simulink model "PMSM_Drive_FastSimulation"  (R2024a)
settings: Solver=ode23t  StartTime=0.0  StopTime=0.2  FixedStep=Ts  RelTol=1e-3  AbsTol=1e-3
PreLoadFcn:
  | % Control parameters
  | Ts = 2e-6;   % Fundamental sample time
  | fsw = 2e3;   % Switching frequency (Hz)
  | fc = fsw*10; % Control loop frequency (Hz)
  | Tsc = 1/fc;  % Control loop sample time
  | 
  | % PMSM parameters
  | PM = 0.03; % Permanent magnet flux linkage
  | Ld = 2e-4;  % d-axis inductance
  | Lq = 2e-4;  % q-axis inductance
  | L0 = 2e-4;  % 0-axis inductance
  | Rs = 0.013; % Stator resistance
  | N = 6; % Number of pole pairs
  | J = 0.2; % Moment of inertia
  | 
  | % Operating and derived limits
  | Imax = 100;  % Max stator current (peak value)
  | Tmax = 1.5*N*PM*Imax; % Max lectromagnetic torque
  | fnom = 100;  % Nominal frequency (Hz)
  | rpm_nom = 60*fnom/N;      % Nominal rotor speed (rpm)
  | omegam_nom = 2*pi*fnom/N; % Nominal mechanical rotor speed
  | Pmax = omegam_nom*Tmax;     % Maximum power
StopFcn:
  | out.SimulationMetadata.TimingInfo
libraries: ee_lib x30, nesl_utility x24, simulink x18, fl_lib x5, slpidlib x3, eePwmGeneratorTwoLevel x3, eeTransforms x2, eeGeneralControl x2, batteryecm_lib x1
(part 3 of 3)

== system PMSM_Drive_FastSimulation/Three-phase inverter/Three-phase inverter (detailed)/IGBT B(L) ==
  Gate Driver : ee_lib/Semiconductors & Converters/Gate Driver  port_option=ee.enum.controlport.ps  uHigh=2.0 V  uLow=0.8 V  uHighValue=0.7  uLowValue=0.3  vHigh=15 V  vLow=0 V  tHigh=1 us  tLow=0 us  parameterization=1  rHigh=10 Ohm  rLow=1 Ohm  tRise=20 ns  tFall=20 ns  cLoad=10 nF  enable_faults=0  t_fault=1 s  fault_type=1  ZonTime_specify=off  ZonTime_priority=None  ZonTime=0 s  ZoffTime_specify=off  ZoffTime_priority=None  ZoffTime=0 s
      settings: InternalSimscapePortConfiguration="{\"Bottom\":[],\"Left\":[{\"id\":\"u\",\"label\":\"u\",\"type\":\"input\"}],\"Right\":[{\"id\":\"G\",\"label\":\"G\",\"type\":\"foundation.electrical.electrical\"},{\"id\":\"S\",\"label\":\"S\",\"type\":\"foundation.electrical.electrical\"}],\"Top\":[]}"
  IGBT : ee_lib/Semiconductors & Converters/N-Channel IGBT  model_type=2  Ices=2 mA  Vces=600 V  Vth=6 V  Vce_sat=2.6 V  Ice_sat=400 A  Vge_sat=10 V  Tmeas=25 degC  Vge_vec=[-3 -2 6 7 8 10 12 15 20] V  Vce_vec=[-1 0 0.5 1 1.5 2 2.5 3 3.5 4] V  T_vec=[25, 125] degC  Ic_mat=[-9.9549e-06 0 0.00047135 0.0005092 0.0005105 0.00051175 0.00051299 0.00051423 0.00051548 0.00051672;-9.9549e-06 0 0.00047135 0.0005092 0.0005105 0.00051175 0.00051299 0.00051423 0.00051548 0.00051672;-9.9549e-06 0 0.00047135 0.0005092 0.0005105 0.00051175 0.00051299 0.00051423 0.00051548 0.00051672;-9.955e-06 0 0.0065225 3.3324 48.154 93.661 105.52 105.72 105.93 106.14;-9.955e-06 0 0.0065235 3.5783 70.264 166.33 252.4 317.67 353.38 357.39;-9.955e-06 0 0.006524 3.7206 89.171 228.09 371.63 511.02 642.69 764.04;-9.9869e-06 0 0.0065242 3.7716 97.793 256.21 424.27 592.92 759.2 921.52;-1.015e-05 0 0.0065243 3.8067 104.52 278.11 464.6 654.37 844.57 1033.9;-1.015e-05 0 0.0065244 3.8324 109.92 295.67 496.54 702.28 909.96 1118.3] A  Ic_mat_3D=zeros(8, 10, 2) A  C_param=1  C_GE=23.7 nF  C_GC=2.7 nF  C_CE=0 nF  C_ies=26.4 nF  C_res=2.7 nF  C_oes=0 nF  C_GE_vec=[ 25 31 26.5 24.9 25 24.9 24.6 24.7 24.8 ] nF  C_GC_vec=[ 55 9 5.5 3.1 2.5 2.1 1.9 1.8 1.7 ] nF  C_Vge_vec=0 V  C_CE_vec=[ 5 11 6.5 4.9 3.5 2.7 2.1 1.7 1.4 ] nF  C_ies_vec=[ 80 40 32 28 27.5 27 26.5 26.5 26.5 ] nF  C_res_vec=[ 55 9 5.5 3.1 2.5 2.1 1.9 1.8 1.7 ] nF  C_oes_vec=[ 60 20 12 8 6 4.8 4 3.5 3.1 ] nF  C_Vce_vec=[ 0 1 2 5 10 15 20 25 30 ] V  charge_linearity_param=1  C_OX=20 nF  V_C_OX=-5 V  TF=0 us  TT=0 us  ec=1  VAF=200 V  RC=0.001 Ohm  RE=0.001 Ohm  RG=0.001 Ohm  BF=50  T_param=1  Ices_T2=100 mA  EG=1.11 eV  Vce_sat_T2=3 V  Tmeas2=125 degC  XTI=3  BEX=-1.5  RG_alpha=0 1/K  Tdevice=25 degC  Tdevice_3D=25 degC  has_thermal_port=0  ig_specify=off  ig_priority=None  ig=0 A  ig_nominal_specify=off  ig_nominal_value=1  ig_nominal_unit=A  ic_specify=off  ic_priority=None  ic=0 A  ic_nominal_specify=off  ic_nominal_value=1  ic_nominal_unit=A  vge_specify=off  vge_priority=None  vge=0 V  vge_nominal_specify=off  vge_nominal_value=1  vge_nominal_unit=V  vce_specify=off  vce_priority=None  vce=0 V  vce_nominal_specify=off  vce_nominal_value=1  vce_nominal_unit=V  v_Cge_specify=off  v_Cge_priority=High  v_Cge=0 V  v_Cge_nominal_specify=off  v_Cge_nominal_value=1  v_Cge_nominal_unit=V  v_Cce_specify=off  v_Cce_priority=High  v_Cce=0 V  v_Cce_nominal_specify=off  v_Cce_nominal_value=1  v_Cce_nominal_unit=V  thermal_network_parameterization=ee.enum.thermalNetworkTopology.junctionCase  Rth=[0, 10] K/W  Rth_Cauer=[1, 3, 10] K/W  Rth_Foster=[4, 6] K/W  thermal_mass_parameterization=ee.enum.thermalNetwork.timeconstant  thermal_mass=[0, 1] J/K  thermal_mass_Cauer=[.1, .3, 1] J/K  thermal_mass_Foster=[1.5, 3] J/K  thermal_time_constant=[0, 10] s  thermal_time_constant_Cauer=[1, 3, 10] s  thermal_time_constant_Foster=[6, 18] s  thermal_mass_initial_temperatures=[25, 25] degC  thermal_mass_initial_temperatures_Cauer=[25, 25, 25] degC  Tvec_initial_Foster=[25, 25, 25, 25] degC  Ic_vec1=[0, 10, 50, 100, 200, 400, 600] A  Vce_vec1=[0, 1.1, 1.3, 1.45, 1.75, 2.25, 2.7] V  Rmiller=0.1 Ohm  Goff=1e-5 1/Ohm  t_on=0.07 us  t_rise=0.7 us  t_off=0.2 us  t_fall=0.5 us  v_meas=300 V  vStartTurnOn_specify=off  vStartTurnOn_priority=None  vStartTurnOn=1 V  tStartTurnOn_specify=off  tStartTurnOn_priority=None  tStartTurnOn=0 s  vStartTurnOff_specify=off  vStartTurnOff_priority=None  vStartTurnOff=0.5 V  tStartTurnOff_specify=off  tStartTurnOff_priority=None  tStartTurnOff=0 s  Tj_vec1=[298.15, 398.15] K  Vce_mat1=[0, 1.1, 1.3, 1.45, 1.75, 2.25, 2.7; 0, 1, 1.15, 1.35, 1.7, 2.35, 3] V  Tj_vec_loss=[298.15, 398.15] K  Ic_vec_loss=[0, 10, 50, 100, 200, 400, 600] A  E_turn_on_mat1=[0, .2, 1, 2, 4, 8, 15; 0, .3, 1.3, 2.5, 5, 11, 18] * 1e-3 J  E_turn_off_mat1=[0, .3, 1.5, 3, 6, 15, 25; 0, .7, 3.3, 6.5, 13, 25, 35] * 1e-3 J  iStartTurnOff_specify=off  iStartTurnOff_priority=None  iStartTurnOff=0 A  Tdevice_specify=off  Tdevice_priority=None
      settings: LogSimulationData=on  InternalSimscapePortConfiguration="{\"Bottom\":[],\"Left\":[{\"id\":\"G\",\"label\":\"\",\"type\":\"foundation.electrical.electrical\"}],\"Right\":[{\"id\":\"C\",\"label\":\"\",\"type\":\"foundation.electrical.electrical\"},{\"id\":\"E\",\"label\":\"\",\"type\":\"foundation.electrical.electrical\"}],\"Top\":[]}"
  + : PMIOPort  Side=Right
  - : PMIOPort  Port=2  Side=Right
  G A(H) : PMIOPort  Port=3  Side=Left
  connections:
  IGBT/RConn1 -- +/RConn1
  -/RConn1 -- IGBT/RConn2 -- Gate Driver/RConn2
  Gate Driver/RConn1 -- IGBT/LConn1
  Gate Driver/LConn1 -- G A(H)/RConn1

== system PMSM_Drive_FastSimulation/Three-phase inverter/Three-phase inverter (detailed)/IGBT C(H) ==
  Gate Driver : ee_lib/Semiconductors & Converters/Gate Driver  port_option=ee.enum.controlport.ps  uHigh=2.0 V  uLow=0.8 V  uHighValue=0.7  uLowValue=0.3  vHigh=15 V  vLow=0 V  tHigh=1 us  tLow=0 us  parameterization=1  rHigh=10 Ohm  rLow=1 Ohm  tRise=20 ns  tFall=20 ns  cLoad=10 nF  enable_faults=0  t_fault=1 s  fault_type=1  ZonTime_specify=off  ZonTime_priority=None  ZonTime=0 s  ZoffTime_specify=off  ZoffTime_priority=None  ZoffTime=0 s
      settings: InternalSimscapePortConfiguration="{\"Bottom\":[],\"Left\":[{\"id\":\"u\",\"label\":\"u\",\"type\":\"input\"}],\"Right\":[{\"id\":\"G\",\"label\":\"G\",\"type\":\"foundation.electrical.electrical\"},{\"id\":\"S\",\"label\":\"S\",\"type\":\"foundation.electrical.electrical\"}],\"Top\":[]}"
  IGBT : ee_lib/Semiconductors & Converters/N-Channel IGBT  model_type=2  Ices=2 mA  Vces=600 V  Vth=6 V  Vce_sat=2.6 V  Ice_sat=400 A  Vge_sat=10 V  Tmeas=25 degC  Vge_vec=[-3 -2 6 7 8 10 12 15 20] V  Vce_vec=[-1 0 0.5 1 1.5 2 2.5 3 3.5 4] V  T_vec=[25, 125] degC  Ic_mat=[-9.9549e-06 0 0.00047135 0.0005092 0.0005105 0.00051175 0.00051299 0.00051423 0.00051548 0.00051672;-9.9549e-06 0 0.00047135 0.0005092 0.0005105 0.00051175 0.00051299 0.00051423 0.00051548 0.00051672;-9.9549e-06 0 0.00047135 0.0005092 0.0005105 0.00051175 0.00051299 0.00051423 0.00051548 0.00051672;-9.955e-06 0 0.0065225 3.3324 48.154 93.661 105.52 105.72 105.93 106.14;-9.955e-06 0 0.0065235 3.5783 70.264 166.33 252.4 317.67 353.38 357.39;-9.955e-06 0 0.006524 3.7206 89.171 228.09 371.63 511.02 642.69 764.04;-9.9869e-06 0 0.0065242 3.7716 97.793 256.21 424.27 592.92 759.2 921.52;-1.015e-05 0 0.0065243 3.8067 104.52 278.11 464.6 654.37 844.57 1033.9;-1.015e-05 0 0.0065244 3.8324 109.92 295.67 496.54 702.28 909.96 1118.3] A  Ic_mat_3D=zeros(8, 10, 2) A  C_param=1  C_GE=23.7 nF  C_GC=2.7 nF  C_CE=0 nF  C_ies=26.4 nF  C_res=2.7 nF  C_oes=0 nF  C_GE_vec=[ 25 31 26.5 24.9 25 24.9 24.6 24.7 24.8 ] nF  C_GC_vec=[ 55 9 5.5 3.1 2.5 2.1 1.9 1.8 1.7 ] nF  C_Vge_vec=0 V  C_CE_vec=[ 5 11 6.5 4.9 3.5 2.7 2.1 1.7 1.4 ] nF  C_ies_vec=[ 80 40 32 28 27.5 27 26.5 26.5 26.5 ] nF  C_res_vec=[ 55 9 5.5 3.1 2.5 2.1 1.9 1.8 1.7 ] nF  C_oes_vec=[ 60 20 12 8 6 4.8 4 3.5 3.1 ] nF  C_Vce_vec=[ 0 1 2 5 10 15 20 25 30 ] V  charge_linearity_param=1  C_OX=20 nF  V_C_OX=-5 V  TF=0 us  TT=0 us  ec=1  VAF=200 V  RC=0.001 Ohm  RE=0.001 Ohm  RG=0.001 Ohm  BF=50  T_param=1  Ices_T2=100 mA  EG=1.11 eV  Vce_sat_T2=3 V  Tmeas2=125 degC  XTI=3  BEX=-1.5  RG_alpha=0 1/K  Tdevice=25 degC  Tdevice_3D=25 degC  has_thermal_port=0  ig_specify=off  ig_priority=None  ig=0 A  ig_nominal_specify=off  ig_nominal_value=1  ig_nominal_unit=A  ic_specify=off  ic_priority=None  ic=0 A  ic_nominal_specify=off  ic_nominal_value=1  ic_nominal_unit=A  vge_specify=off  vge_priority=None  vge=0 V  vge_nominal_specify=off  vge_nominal_value=1  vge_nominal_unit=V  vce_specify=off  vce_priority=None  vce=0 V  vce_nominal_specify=off  vce_nominal_value=1  vce_nominal_unit=V  v_Cge_specify=off  v_Cge_priority=High  v_Cge=0 V  v_Cge_nominal_specify=off  v_Cge_nominal_value=1  v_Cge_nominal_unit=V  v_Cce_specify=off  v_Cce_priority=High  v_Cce=0 V  v_Cce_nominal_specify=off  v_Cce_nominal_value=1  v_Cce_nominal_unit=V  thermal_network_parameterization=ee.enum.thermalNetworkTopology.junctionCase  Rth=[0, 10] K/W  Rth_Cauer=[1, 3, 10] K/W  Rth_Foster=[4, 6] K/W  thermal_mass_parameterization=ee.enum.thermalNetwork.timeconstant  thermal_mass=[0, 1] J/K  thermal_mass_Cauer=[.1, .3, 1] J/K  thermal_mass_Foster=[1.5, 3] J/K  thermal_time_constant=[0, 10] s  thermal_time_constant_Cauer=[1, 3, 10] s  thermal_time_constant_Foster=[6, 18] s  thermal_mass_initial_temperatures=[25, 25] degC  thermal_mass_initial_temperatures_Cauer=[25, 25, 25] degC  Tvec_initial_Foster=[25, 25, 25, 25] degC  Ic_vec1=[0, 10, 50, 100, 200, 400, 600] A  Vce_vec1=[0, 1.1, 1.3, 1.45, 1.75, 2.25, 2.7] V  Rmiller=0.1 Ohm  Goff=1e-5 1/Ohm  t_on=0.07 us  t_rise=0.7 us  t_off=0.2 us  t_fall=0.5 us  v_meas=300 V  vStartTurnOn_specify=off  vStartTurnOn_priority=None  vStartTurnOn=1 V  tStartTurnOn_specify=off  tStartTurnOn_priority=None  tStartTurnOn=0 s  vStartTurnOff_specify=off  vStartTurnOff_priority=None  vStartTurnOff=0.5 V  tStartTurnOff_specify=off  tStartTurnOff_priority=None  tStartTurnOff=0 s  Tj_vec1=[298.15, 398.15] K  Vce_mat1=[0, 1.1, 1.3, 1.45, 1.75, 2.25, 2.7; 0, 1, 1.15, 1.35, 1.7, 2.35, 3] V  Tj_vec_loss=[298.15, 398.15] K  Ic_vec_loss=[0, 10, 50, 100, 200, 400, 600] A  E_turn_on_mat1=[0, .2, 1, 2, 4, 8, 15; 0, .3, 1.3, 2.5, 5, 11, 18] * 1e-3 J  E_turn_off_mat1=[0, .3, 1.5, 3, 6, 15, 25; 0, .7, 3.3, 6.5, 13, 25, 35] * 1e-3 J  iStartTurnOff_specify=off  iStartTurnOff_priority=None  iStartTurnOff=0 A  Tdevice_specify=off  Tdevice_priority=None
      settings: LogSimulationData=on  InternalSimscapePortConfiguration="{\"Bottom\":[],\"Left\":[{\"id\":\"G\",\"label\":\"\",\"type\":\"foundation.electrical.electrical\"}],\"Right\":[{\"id\":\"C\",\"label\":\"\",\"type\":\"foundation.electrical.electrical\"},{\"id\":\"E\",\"label\":\"\",\"type\":\"foundation.electrical.electrical\"}],\"Top\":[]}"
  + : PMIOPort  Side=Right
  - : PMIOPort  Port=2  Side=Right
  G A(H) : PMIOPort  Port=3  Side=Left
  connections:
  IGBT/RConn1 -- +/RConn1
  -/RConn1 -- IGBT/RConn2 -- Gate Driver/RConn2
  Gate Driver/RConn1 -- IGBT/LConn1
  Gate Driver/LConn1 -- G A(H)/RConn1

== system PMSM_Drive_FastSimulation/Three-phase inverter/Three-phase inverter (detailed)/IGBT C(L) ==
  Gate Driver : ee_lib/Semiconductors & Converters/Gate Driver  port_option=ee.enum.controlport.ps  uHigh=2.0 V  uLow=0.8 V  uHighValue=0.7  uLowValue=0.3  vHigh=15 V  vLow=0 V  tHigh=1 us  tLow=0 us  parameterization=1  rHigh=10 Ohm  rLow=1 Ohm  tRise=20 ns  tFall=20 ns  cLoad=10 nF  enable_faults=0  t_fault=1 s  fault_type=1  ZonTime_specify=off  ZonTime_priority=None  ZonTime=0 s  ZoffTime_specify=off  ZoffTime_priority=None  ZoffTime=0 s
      settings: InternalSimscapePortConfiguration="{\"Bottom\":[],\"Left\":[{\"id\":\"u\",\"label\":\"u\",\"type\":\"input\"}],\"Right\":[{\"id\":\"G\",\"label\":\"G\",\"type\":\"foundation.electrical.electrical\"},{\"id\":\"S\",\"label\":\"S\",\"type\":\"foundation.electrical.electrical\"}],\"Top\":[]}"
  IGBT : ee_lib/Semiconductors & Converters/N-Channel IGBT  model_type=2  Ices=2 mA  Vces=600 V  Vth=6 V  Vce_sat=2.6 V  Ice_sat=400 A  Vge_sat=10 V  Tmeas=25 degC  Vge_vec=[-3 -2 6 7 8 10 12 15 20] V  Vce_vec=[-1 0 0.5 1 1.5 2 2.5 3 3.5 4] V  T_vec=[25, 125] degC  Ic_mat=[-9.9549e-06 0 0.00047135 0.0005092 0.0005105 0.00051175 0.00051299 0.00051423 0.00051548 0.00051672;-9.9549e-06 0 0.00047135 0.0005092 0.0005105 0.00051175 0.00051299 0.00051423 0.00051548 0.00051672;-9.9549e-06 0 0.00047135 0.0005092 0.0005105 0.00051175 0.00051299 0.00051423 0.00051548 0.00051672;-9.955e-06 0 0.0065225 3.3324 48.154 93.661 105.52 105.72 105.93 106.14;-9.955e-06 0 0.0065235 3.5783 70.264 166.33 252.4 317.67 353.38 357.39;-9.955e-06 0 0.006524 3.7206 89.171 228.09 371.63 511.02 642.69 764.04;-9.9869e-06 0 0.0065242 3.7716 97.793 256.21 424.27 592.92 759.2 921.52;-1.015e-05 0 0.0065243 3.8067 104.52 278.11 464.6 654.37 844.57 1033.9;-1.015e-05 0 0.0065244 3.8324 109.92 295.67 496.54 702.28 909.96 1118.3] A  Ic_mat_3D=zeros(8, 10, 2) A  C_param=1  C_GE=23.7 nF  C_GC=2.7 nF  C_CE=0 nF  C_ies=26.4 nF  C_res=2.7 nF  C_oes=0 nF  C_GE_vec=[ 25 31 26.5 24.9 25 24.9 24.6 24.7 24.8 ] nF  C_GC_vec=[ 55 9 5.5 3.1 2.5 2.1 1.9 1.8 1.7 ] nF  C_Vge_vec=0 V  C_CE_vec=[ 5 11 6.5 4.9 3.5 2.7 2.1 1.7 1.4 ] nF  C_ies_vec=[ 80 40 32 28 27.5 27 26.5 26.5 26.5 ] nF  C_res_vec=[ 55 9 5.5 3.1 2.5 2.1 1.9 1.8 1.7 ] nF  C_oes_vec=[ 60 20 12 8 6 4.8 4 3.5 3.1 ] nF  C_Vce_vec=[ 0 1 2 5 10 15 20 25 30 ] V  charge_linearity_param=1  C_OX=20 nF  V_C_OX=-5 V  TF=0 us  TT=0 us  ec=1  VAF=200 V  RC=0.001 Ohm  RE=0.001 Ohm  RG=0.001 Ohm  BF=50  T_param=1  Ices_T2=100 mA  EG=1.11 eV  Vce_sat_T2=3 V  Tmeas2=125 degC  XTI=3  BEX=-1.5  RG_alpha=0 1/K  Tdevice=25 degC  Tdevice_3D=25 degC  has_thermal_port=0  ig_specify=off  ig_priority=None  ig=0 A  ig_nominal_specify=off  ig_nominal_value=1  ig_nominal_unit=A  ic_specify=off  ic_priority=None  ic=0 A  ic_nominal_specify=off  ic_nominal_value=1  ic_nominal_unit=A  vge_specify=off  vge_priority=None  vge=0 V  vge_nominal_specify=off  vge_nominal_value=1  vge_nominal_unit=V  vce_specify=off  vce_priority=None  vce=0 V  vce_nominal_specify=off  vce_nominal_value=1  vce_nominal_unit=V  v_Cge_specify=off  v_Cge_priority=High  v_Cge=0 V  v_Cge_nominal_specify=off  v_Cge_nominal_value=1  v_Cge_nominal_unit=V  v_Cce_specify=off  v_Cce_priority=High  v_Cce=0 V  v_Cce_nominal_specify=off  v_Cce_nominal_value=1  v_Cce_nominal_unit=V  thermal_network_parameterization=ee.enum.thermalNetworkTopology.junctionCase  Rth=[0, 10] K/W  Rth_Cauer=[1, 3, 10] K/W  Rth_Foster=[4, 6] K/W  thermal_mass_parameterization=ee.enum.thermalNetwork.timeconstant  thermal_mass=[0, 1] J/K  thermal_mass_Cauer=[.1, .3, 1] J/K  thermal_mass_Foster=[1.5, 3] J/K  thermal_time_constant=[0, 10] s  thermal_time_constant_Cauer=[1, 3, 10] s  thermal_time_constant_Foster=[6, 18] s  thermal_mass_initial_temperatures=[25, 25] degC  thermal_mass_initial_temperatures_Cauer=[25, 25, 25] degC  Tvec_initial_Foster=[25, 25, 25, 25] degC  Ic_vec1=[0, 10, 50, 100, 200, 400, 600] A  Vce_vec1=[0, 1.1, 1.3, 1.45, 1.75, 2.25, 2.7] V  Rmiller=0.1 Ohm  Goff=1e-5 1/Ohm  t_on=0.07 us  t_rise=0.7 us  t_off=0.2 us  t_fall=0.5 us  v_meas=300 V  vStartTurnOn_specify=off  vStartTurnOn_priority=None  vStartTurnOn=1 V  tStartTurnOn_specify=off  tStartTurnOn_priority=None  tStartTurnOn=0 s  vStartTurnOff_specify=off  vStartTurnOff_priority=None  vStartTurnOff=0.5 V  tStartTurnOff_specify=off  tStartTurnOff_priority=None  tStartTurnOff=0 s  Tj_vec1=[298.15, 398.15] K  Vce_mat1=[0, 1.1, 1.3, 1.45, 1.75, 2.25, 2.7; 0, 1, 1.15, 1.35, 1.7, 2.35, 3] V  Tj_vec_loss=[298.15, 398.15] K  Ic_vec_loss=[0, 10, 50, 100, 200, 400, 600] A  E_turn_on_mat1=[0, .2, 1, 2, 4, 8, 15; 0, .3, 1.3, 2.5, 5, 11, 18] * 1e-3 J  E_turn_off_mat1=[0, .3, 1.5, 3, 6, 15, 25; 0, .7, 3.3, 6.5, 13, 25, 35] * 1e-3 J  iStartTurnOff_specify=off  iStartTurnOff_priority=None  iStartTurnOff=0 A  Tdevice_specify=off  Tdevice_priority=None
      settings: LogSimulationData=on  InternalSimscapePortConfiguration="{\"Bottom\":[],\"Left\":[{\"id\":\"G\",\"label\":\"\",\"type\":\"foundation.electrical.electrical\"}],\"Right\":[{\"id\":\"C\",\"label\":\"\",\"type\":\"foundation.electrical.electrical\"},{\"id\":\"E\",\"label\":\"\",\"type\":\"foundation.electrical.electrical\"}],\"Top\":[]}"
  + : PMIOPort  Side=Right
  - : PMIOPort  Port=2  Side=Right
  G A(H) : PMIOPort  Port=3  Side=Left
  connections:
  Gate Driver/LConn1 -- G A(H)/RConn1
  Gate Driver/RConn1 -- IGBT/LConn1
  Gate Driver/RConn2 -- IGBT/RConn2 -- -/RConn1
  IGBT/RConn1 -- +/RConn1

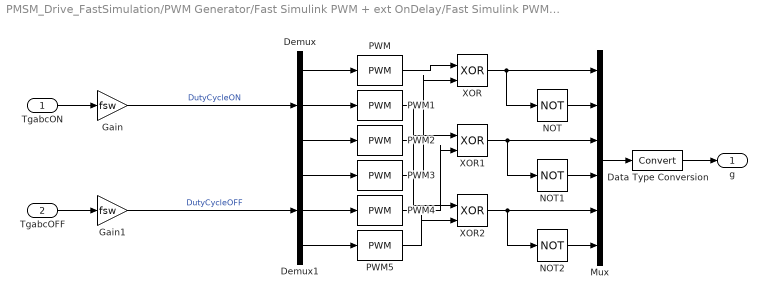
== system PMSM_Drive_FastSimulation/PWM Generator/Fast Simulink PWM + ext OnDelay/Fast Simulink PWM/Fast Simulink PWM Generator ==
  TgabcON : Inport
  TgabcOFF : Inport  Port=2
  Data Type Conversion : DataTypeConversion  SaturateOnIntegerOverflow=off  RndMeth=Floor
  Demux : Demux  Outputs=3
  Demux1 : Demux  Outputs=3
  Gain : Gain  Gain=fsw
  Gain1 : Gain  Gain=fsw
  Mux : Mux  Inputs=6
  NOT : Logic  Operator=NOT  IconShape=distinctive  AllPortsSameDT=off  OutDataTypeStr=boolean
  NOT1 : Logic  Operator=NOT  IconShape=distinctive  AllPortsSameDT=off  OutDataTypeStr=boolean
  NOT2 : Logic  Operator=NOT  IconShape=distinctive  AllPortsSameDT=off  OutDataTypeStr=boolean
  PWM{,1..5} (6 alike) : simulink/Discontinuities/PWM  DisableCoverage=on  Period=1/fsw  InitialDelay=0  DisallowZeroDutyCycle=off  RunAtFixedTimeIntervals=off  SampleTime=Ts
  XOR : Logic  Operator=XOR  IconShape=distinctive  AllPortsSameDT=off  OutDataTypeStr=boolean
  XOR1 : Logic  Operator=XOR  IconShape=distinctive  AllPortsSameDT=off  OutDataTypeStr=boolean
  XOR2 : Logic  Operator=XOR  IconShape=distinctive  AllPortsSameDT=off  OutDataTypeStr=boolean
  g : Outport
  wires:
  Mux/1 -> Data Type Conversion/1
  Demux1/3 -> PWM5/1
  Demux1/2 -> PWM4/1
  Demux1/1 -> PWM3/1
  Demux/3 -> PWM2/1
  Demux/2 -> PWM1/1
  Demux/1 -> PWM/1
  TgabcOFF/1 -> Gain1/1
  TgabcON/1 -> Gain/1
  PWM/1 -> XOR/1
  PWM3/1 -> XOR/2
  PWM1/1 -> XOR1/1
  PWM4/1 -> XOR1/2
  PWM2/1 -> XOR2/1
  PWM5/1 -> XOR2/2
  XOR/1 -> NOT/1, Mux/1
  XOR2/1 -> NOT2/1, Mux/5
  XOR1/1 -> NOT1/1, Mux/3
  NOT/1 -> Mux/2
  NOT1/1 -> Mux/4
  NOT2/1 -> Mux/6
  Data Type Conversion/1 -> g/1
  Gain/1 -> Demux/1  "DutyCycleON"
  Gain1/1 -> Demux1/1  "DutyCycleOFF"

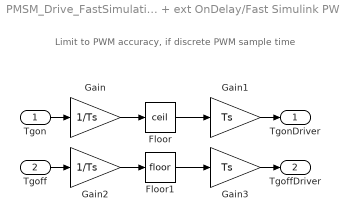
== system PMSM_Drive_FastSimulation/PWM Generator/Fast Simulink PWM + ext OnDelay/Fast Simulink PWM/synchronous PWM ==
  note: Limit to PWM accuracy, if discrete PWM sample time
  Tgon : Inport
  Tgoff : Inport  Port=2
  Floor : Rounding  Operator=ceil
  Floor1 : Rounding
  Gain : Gain  Gain=1/Ts
  Gain1 : Gain  Gain=Ts
  Gain2 : Gain  Gain=1/Ts
  Gain3 : Gain  Gain=Ts
  TgonDriver : Outport
  TgoffDriver : Outport  Port=2
  wires:
  Floor1/1 -> Gain3/1
  Gain1/1 -> TgonDriver/1
  Gain/1 -> Floor/1
  Gain2/1 -> Floor1/1
  Floor/1 -> Gain1/1
  Tgoff/1 -> Gain2/1
  Gain3/1 -> TgoffDriver/1
  Tgon/1 -> Gain/1

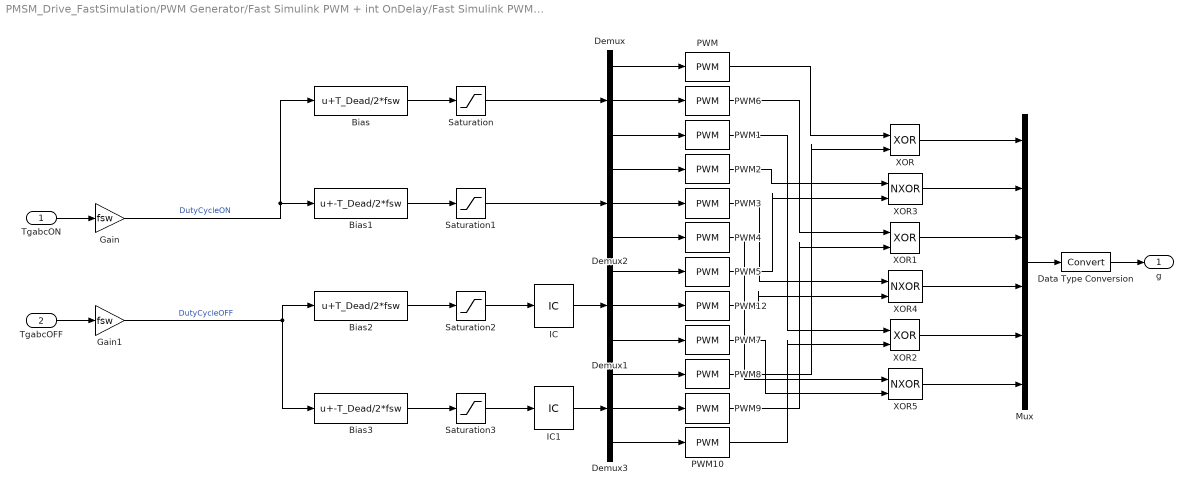
== system PMSM_Drive_FastSimulation/PWM Generator/Fast Simulink PWM + int OnDelay/Fast Simulink PWM/Fast Simulink PWM Generator HL Dead Time ==
  TgabcON : Inport
  TgabcOFF : Inport  Port=2
  Bias : Bias  Bias=T_Dead/2*fsw  SaturateOnIntegerOverflow=off
  Bias1 : Bias  Bias=-T_Dead/2*fsw  SaturateOnIntegerOverflow=off
  Bias2 : Bias  Bias=T_Dead/2*fsw  SaturateOnIntegerOverflow=off
  Bias3 : Bias  Bias=-T_Dead/2*fsw  SaturateOnIntegerOverflow=off
  Data Type Conversion : DataTypeConversion  SaturateOnIntegerOverflow=off  RndMeth=Floor
  Demux{,1..3} (4 alike) : Demux  Outputs=3
  Gain : Gain  Gain=fsw
  Gain1 : Gain  Gain=fsw
  IC : InitialCondition  Value=[0 0 0]
  IC1 : InitialCondition  Value=[0 0 0]
  Mux : Mux  Inputs=6
  PWM{,1..10,12} (12 alike) : simulink/Discontinuities/PWM  DisableCoverage=on  Period=1/fsw  InitialDelay=0  DisallowZeroDutyCycle=off  RunAtFixedTimeIntervals=off  SampleTime=Ts
  Saturation : Saturate  UpperLimit=1/2  LowerLimit=0
  Saturation1 : Saturate  UpperLimit=1/2  LowerLimit=0
  Saturation2 : Saturate  UpperLimit=1  LowerLimit=1/2
  Saturation3 : Saturate  UpperLimit=1  LowerLimit=1/2
  XOR : Logic  Operator=XOR  IconShape=distinctive  AllPortsSameDT=off  OutDataTypeStr=boolean
  XOR1 : Logic  Operator=XOR  IconShape=distinctive  AllPortsSameDT=off  OutDataTypeStr=boolean
  XOR2 : Logic  Operator=XOR  IconShape=distinctive  AllPortsSameDT=off  OutDataTypeStr=boolean
  XOR3 : Logic  Operator=NXOR  IconShape=distinctive  AllPortsSameDT=off  OutDataTypeStr=boolean
  XOR4 : Logic  Operator=NXOR  IconShape=distinctive  AllPortsSameDT=off  OutDataTypeStr=boolean
  XOR5 : Logic  Operator=NXOR  IconShape=distinctive  AllPortsSameDT=off  OutDataTypeStr=boolean
  g : Outport
  wires:
  IC/1 -> Demux1/1
  IC1/1 -> Demux3/1
  Saturation3/1 -> IC1/1
  Saturation2/1 -> IC/1
  Saturation1/1 -> Demux2/1
  Saturation/1 -> Demux/1
  PWM7/1 -> XOR5/2
  PWM4/1 -> XOR5/1
  PWM12/1 -> XOR4/2
  PWM3/1 -> XOR4/1
  PWM2/1 -> XOR3/1
  PWM10/1 -> XOR2/2
  PWM1/1 -> XOR2/1
  PWM9/1 -> XOR1/2
  PWM6/1 -> XOR1/1
  PWM/1 -> XOR/1
  PWM8/1 -> XOR/2
  PWM5/1 -> XOR3/2
  Bias3/1 -> Saturation3/1
  Demux3/3 -> PWM10/1
  Demux3/2 -> PWM9/1
  Demux3/1 -> PWM8/1
  Demux1/3 -> PWM7/1
  Demux1/2 -> PWM12/1
  Demux1/1 -> PWM5/1
  Bias1/1 -> Saturation1/1
  Demux2/3 -> PWM4/1
  Demux2/2 -> PWM3/1
  Demux2/1 -> PWM2/1
  Demux/3 -> PWM1/1
  Demux/2 -> PWM6/1
  Demux/1 -> PWM/1
  Bias2/1 -> Saturation2/1
  Bias/1 -> Saturation/1
  Mux/1 -> Data Type Conversion/1
  TgabcOFF/1 -> Gain1/1
  TgabcON/1 -> Gain/1
  XOR/1 -> Mux/1
  XOR2/1 -> Mux/5
  XOR1/1 -> Mux/3
  XOR3/1 -> Mux/2
  XOR4/1 -> Mux/4
  XOR5/1 -> Mux/6
  Data Type Conversion/1 -> g/1
  Gain/1 -> Bias/1, Bias1/1  "DutyCycleON"
  Gain1/1 -> Bias2/1, Bias3/1  "DutyCycleOFF"

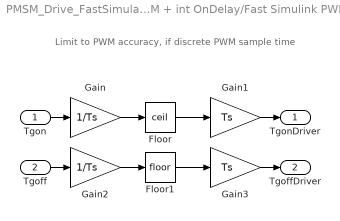
== system PMSM_Drive_FastSimulation/PWM Generator/Fast Simulink PWM + int OnDelay/Fast Simulink PWM/synchronous PWM ==
  note: Limit to PWM accuracy, if discrete PWM sample time
  Tgon : Inport
  Tgoff : Inport  Port=2
  Floor : Rounding  Operator=ceil
  Floor1 : Rounding
  Gain : Gain  Gain=1/Ts
  Gain1 : Gain  Gain=Ts
  Gain2 : Gain  Gain=1/Ts
  Gain3 : Gain  Gain=Ts
  TgonDriver : Outport
  TgoffDriver : Outport  Port=2
  wires:
  Tgon/1 -> Gain/1
  Gain3/1 -> TgoffDriver/1
  Tgoff/1 -> Gain2/1
  Floor/1 -> Gain1/1
  Gain2/1 -> Floor1/1
  Gain/1 -> Floor/1
  Gain1/1 -> TgonDriver/1
  Floor1/1 -> Gain3/1
